simulink model "ISRTest2"  (Simulink 6.6)
settings: Solver=ode3  StartTime=0.0  StopTime=time(end)  FixedStep=0.01  RelTol=1e-3
values from neighbouring files (symbols this model uses):
  apSampleTime = 0.01    [Load_Replay.m]    (also in loadReplayMay2013.m; loadTuneRollReplay_May2013.m)
undefined symbols (not defined in the file or in its folder): bankCommandLimit, fOrderingInOut, ISA_g, maxAcc, maxEta
libraries: simulink x14, aerolibconvert2 x11, dsPICdrivers x7, SLUGS_Library x3, dspmtrx3 x2, aerolibutil x1
(part 2 of 2)

== system ISRTest2/Get 2D Groundspeed/Norm/Subsystem1 ==
  x : Inport
  C Function Call : S-Function  Tag=dsPIC_dsPIC_CFunctionCall  FunctionName=dsPIC_C_function_Call  Parameters=INPUT_SIZE,OUTPUT_SIZE,InputType,OutputType,SampleTime,fOrderingInOut  mask(C Function Call){fctName='mySqrt', INPUT_SIZE=1, INPUT1=real32, INPUT2=--, INPUT3=--, OUTPUT_SIZE=1, OUTPUT1=real32, SampleTime=-1, InputType=[ 7 ], OutputType=[ 7 ], FctDeclaration=extern real32_T mySqrt(real32_T u1);, FctCall=%y1 = mySqrt(%u1);, OrderingInOutPopup=None}
      mask prompts: fctName "Function Name"; INPUT_SIZE "Global Input Size"; INPUT1 "Input 1"; INPUT2 "Input 2"; INPUT3 "Input 3"; OUTPUT_SIZE "Output size"; OUTPUT1 "Output type"; InputType "NbrInput"; OutputType "NbrOutput"; FctDeclaration "Function Declaration :"; FctCall "Function Call :"; OrderingInOutPopup "Block Ordering Input / Output"
      mask help: call user defined C function
      mask init:
      | dsPIC_C_function_Call_callback();
      mask Help: http://www.kerhuel.eu/wiki/index.php5?title=Block/C_Function_Call#1
      mask StyleString: edit,edit,popup(--|int8|uint8|int16|uint16|int32|uint32|real32|real64),popup(--|int8|uint8|int16|uint16|int32|uint32|real32|real64),popup(--|int8|uint8|int16|uint16|int32|uint32|real32|real64),edit,popup(--|int8|uint8|int16|uint16|int32|uint32|real32|real64),edit,edit,edit,edit,edit,popup(None|Input|Output|Input & Output)
      mask CallbackString:
      | dsPIC_C_function_Call_callback();|dsPIC_C_function_Call_callback();|dsPIC_C_function_Call_callback();|dsPIC_C_function_Call_callback();
      | |dsPIC_C_function_Call_callback();|dsPIC_C_function_Call_callback();|dsPIC_C_function_Call_callback();|dsPIC_C_function_Call_callback();|||% for information only|% for information only|
      mask Display:
      | fprintf('C function call\nmySqrt');
      | port_label('input',1,' u1');
      | port_label('output',1,'y');
  Environment Controller : Subsystem  mask(Environment Controller){}
      mask help: Output the simulation (Sim) or Real-Time Workshop (RTW) port depending on the current environment. With optimizations enabled, unnecessary blocks leading to the unused port are not executed. Both input signals must be the same width.
      mask init:
      | switch_mode = rtwenvironmentmode(bdroot(gcbh));
  Math Function1 : Math  Operator=sqrt  SaturateOnIntegerOverflow=on
  negprotect : Stateflow chart
  sqrt(x) : Outport
  wires:
  C Function Call/1 -> Environment Controller/2(RTW)
  Math Function1/1 -> Environment Controller/1(Sim)
  Environment Controller/1(Out) -> sqrt(x)/1
  negprotect/1(zpVal) -> C Function Call/1, Math Function1/1
  x/1 -> negprotect/1(val)

== system ISRTest2/L2+/Get Sin, Cos eta/2D Dot Product  ==
  Vxyz : Inport
  L2_vec : Inport  Port=2
  Demux : Demux  Outputs=3
  Demux1 : Demux  Outputs=3
  Product : Product  RndMeth=Zero
  Product1 : Product  RndMeth=Zero
  Subtract : Sum  Inputs=2  OutScaling=2^-10
  Terminator : Terminator
  Terminator1 : Terminator
  2D _dot : Outport
  wires:
  Vxyz/1 -> Demux/1
  Subtract/1 -> 2D _dot/1
  L2_vec/1 -> Demux1/1
  Product1/1 -> Subtract/2
  Product/1 -> Subtract/1
  Demux1/3 -> Terminator1/1
  Demux/3 -> Terminator/1
  Demux1/1 -> Product/1
  Demux/1 -> Product/2
  Demux1/2 -> Product1/1
  Demux/2 -> Product1/2

== system ISRTest2/L2+/Get Sin, Cos eta/Get  Groundspeed ==
  L2_vec : Inport  SampleTime=apSampleTime
  Norm : Subsystem
  Zero out Z1 : Stateflow chart
  |L2| : Outport
  wires:
  L2_vec/1 -> Zero out Z1/1(Pin)
  Zero out Z1/1(P) -> Norm/1(Vector)
  Norm/1(Norm) -> |L2|/1

== system ISRTest2/L2+/Get Sin, Cos eta/Get ZProd ==
  L2_vec : Inport
  Vxyz : Inport  Port=2
  Demux : Demux  Outputs=3
  Demux1 : Demux  Outputs=3
  Product : Product  RndMeth=Zero
  Product1 : Product  RndMeth=Zero
  Subtract : Sum  Inputs=+-  OutScaling=2^-10
  Terminator : Terminator
  Terminator1 : Terminator
  Z_prod : Outport
  wires:
  Demux/3 -> Terminator/1
  Demux1/3 -> Terminator1/1
  Demux/1 -> Product/2
  Demux1/2 -> Product/1
  Demux/2 -> Product1/2
  Demux1/1 -> Product1/1
  Product/1 -> Subtract/1
  Product1/1 -> Subtract/2
  L2_vec/1 -> Demux1/1
  Subtract/1 -> Z_prod/1
  Vxyz/1 -> Demux/1

== system ISRTest2/L2+/Subsystem/Subsystem2 ==
  x : Inport
  C Function Call : S-Function  Tag=dsPIC_dsPIC_CFunctionCall  AncestorBlock=dsPICdrivers/OTHERS/C Function Call  FunctionName=dsPIC_C_function_Call  Parameters=INPUT_SIZE,OUTPUT_SIZE,InputType,OutputType,SampleTime,fOrderingInOut  mask(C Function Call){fctName='myAtan', INPUT_SIZE=1, INPUT1=real32, INPUT2=--, INPUT3=--, OUTPUT_SIZE=1, OUTPUT1=real32, SampleTime=-1, InputType=[ 7 ], OutputType=[ 7 ], FctDeclaration=extern real32_T myAtan(real32_T u1);, FctCall=%y1 = myAtan(%u1);, OrderingInOutPopup=None}
      mask prompts: fctName "Function Name"; INPUT_SIZE "Global Input Size"; INPUT1 "Input 1"; INPUT2 "Input 2"; INPUT3 "Input 3"; OUTPUT_SIZE "Output size"; OUTPUT1 "Output type"; InputType "NbrInput"; OutputType "NbrOutput"; FctDeclaration "Function Declaration :"; FctCall "Function Call :"; OrderingInOutPopup "Block Ordering Input / Output"
      mask help: call user defined C function
      mask init:
      | dsPIC_C_function_Call_callback();
      mask Help: http://www.kerhuel.eu/wiki/index.php5?title=Block/C_Function_Call#1
      mask StyleString: edit,edit,popup(--|int8|uint8|int16|uint16|int32|uint32|real32|real64),popup(--|int8|uint8|int16|uint16|int32|uint32|real32|real64),popup(--|int8|uint8|int16|uint16|int32|uint32|real32|real64),edit,popup(--|int8|uint8|int16|uint16|int32|uint32|real32|real64),edit,edit,edit,edit,edit,popup(None|Input|Output|Input & Output)
      mask CallbackString:
      | dsPIC_C_function_Call_callback();|dsPIC_C_function_Call_callback();|dsPIC_C_function_Call_callback();|dsPIC_C_function_Call_callback();
      | |dsPIC_C_function_Call_callback();|dsPIC_C_function_Call_callback();|dsPIC_C_function_Call_callback();|dsPIC_C_function_Call_callback();|||% for information only|% for information only|
      mask Display:
      | fprintf('C function call\nmyAtan');
      | port_label('input',1,' u1');
      | port_label('output',1,'y');
  Environment Controller : Subsystem  AncestorBlock=|  mask(Environment Controller){}
      | simulink/Signal
      | Routing/Environment
      | Controller
      mask help: Output the simulation (Sim) or Real-Time Workshop (RTW) port depending on the current environment. With optimizations enabled, unnecessary blocks leading to the unused port are not executed. Both input signals must be the same width.
      mask init:
      | switch_mode = rtwenvironmentmode(bdroot(gcbh));
  Trigonometric Function : Trigonometry  Operator=atan
  atan(x) : Outport
  wires:
  x/1 -> C Function Call/1, Trigonometric Function/1
  Trigonometric Function/1 -> Environment Controller/1(Sim)
  C Function Call/1 -> Environment Controller/2(RTW)
  Environment Controller/1(Out) -> atan(x)/1

== system ISRTest2/L2+/Subsystem4/Environment Controller ==
  Sim : Inport
  RTW : Inport  Port=2
  Environment Switch : Switch  Criteria=u2 ~= 0  ZeroCross=off  InputSameDT=on
  Numerical Unity : SignalConversion  ConversionOutput=Bus copy
  Switch Control : Constant  Value=switch_mode  OutDataTypeMode=boolean
  Out : Outport
  wires:
  Numerical Unity/1 -> Out/1
  RTW/1 -> Environment Switch/3
  Environment Switch/1 -> Numerical Unity/1
  Switch Control/1 -> Environment Switch/2
  Sim/1 -> Environment Switch/1

== system ISRTest2/Point  Surveillance/P2CC Data/Norm1 ==
  Vector : Inport
  Subsystem1 : Subsystem  AncestorBlock=SLUGS_Library/Subsystem1
  Subsystem3 : Subsystem  AncestorBlock=SLUGS_Library/Subsystem3
  Norm : Outport
  wires:
  Subsystem3/1(x dot y) -> Subsystem1/1(x)
  Vector/1 -> Subsystem3/2(y), Subsystem3/1(x)
  Subsystem1/1(sqrt(x)) -> Norm/1

== system ISRTest2/Point  Surveillance/P2CC Data/Subsystem10 ==
  x : Inport
  Trigonometric Function : Trigonometry  Operator=acos
  acos(x) : Outport
  wires:
  x/1 -> Trigonometric Function/1
  Trigonometric Function/1 -> acos(x)/1

== system ISRTest2/Point  Surveillance/P2CC Data/Subsystem4 ==
  x : Inport
  y : Inport  Port=2
  Trigonometric Function : Trigonometry  Operator=atan2
  atan2(x,y) : Outport
  wires:
  Trigonometric Function/1 -> atan2(x,y)/1
  y/1 -> Trigonometric Function/2
  x/1 -> Trigonometric Function/1

== system ISRTest2/Camera Track/Norm/Subsystem1/Environment Controller ==
  Sim : Inport
  RTW : Inport  Port=2
  Environment Switch : Switch  Criteria=u2 ~= 0  ZeroCross=off  InputSameDT=on
  Numerical Unity : SignalConversion  ConversionOutput=Bus copy
  Switch Control : Constant  Value=switch_mode  OutDataTypeMode=boolean
  Out : Outport
  wires:
  Numerical Unity/1 -> Out/1
  RTW/1 -> Environment Switch/3
  Environment Switch/1 -> Numerical Unity/1
  Switch Control/1 -> Environment Switch/2
  Sim/1 -> Environment Switch/1

== system ISRTest2/Camera Track/Norm1/Subsystem1/Environment Controller ==
  Sim : Inport
  RTW : Inport  Port=2
  Environment Switch : Switch  Criteria=u2 ~= 0  ZeroCross=off  InputSameDT=on
  Numerical Unity : SignalConversion  ConversionOutput=Bus copy
  Switch Control : Constant  Value=switch_mode  OutDataTypeMode=boolean
  Out : Outport
  wires:
  Sim/1 -> Environment Switch/1
  Switch Control/1 -> Environment Switch/2
  Environment Switch/1 -> Numerical Unity/1
  RTW/1 -> Environment Switch/3
  Numerical Unity/1 -> Out/1

== system ISRTest2/Get 2D Groundspeed/Norm/Subsystem1/Environment Controller ==
  Sim : Inport
  RTW : Inport  Port=2
  Environment Switch : Switch  Criteria=u2 ~= 0  ZeroCross=off  InputSameDT=on
  Numerical Unity : SignalConversion  ConversionOutput=Bus copy
  Switch Control : Constant  Value=switch_mode  OutDataTypeMode=boolean
  Out : Outport
  wires:
  Sim/1 -> Environment Switch/1
  Switch Control/1 -> Environment Switch/2
  Environment Switch/1 -> Numerical Unity/1
  RTW/1 -> Environment Switch/3
  Numerical Unity/1 -> Out/1

== system ISRTest2/L2+/Get Sin, Cos eta/Get  Groundspeed/Norm ==
  Vector : Inport
  Subsystem1 : Subsystem  AncestorBlock=SLUGS_Library/Subsystem1
  Subsystem3 : SLUGS_Library/Subsystem3  SystemSampleTime=-1
  Norm : Outport
  wires:
  Subsystem1/1(sqrt(x)) -> Norm/1
  Vector/1 -> Subsystem3/1, Subsystem3/2
  Subsystem3/1 -> Subsystem1/1(x)

== system ISRTest2/L2+/Subsystem/Subsystem2/Environment Controller ==
  Sim : Inport
  RTW : Inport  Port=2
  Environment Switch : Switch  Criteria=u2 ~= 0  ZeroCross=off  InputSameDT=on
  Numerical Unity : SignalConversion  ConversionOutput=Bus copy
  Switch Control : Constant  Value=switch_mode  OutDataTypeMode=boolean
  Out : Outport
  wires:
  Numerical Unity/1 -> Out/1
  RTW/1 -> Environment Switch/3
  Environment Switch/1 -> Numerical Unity/1
  Switch Control/1 -> Environment Switch/2
  Sim/1 -> Environment Switch/1

== system ISRTest2/Point  Surveillance/P2CC Data/Norm1/Subsystem1 ==
  x : Inport
  Math Function : Math  Operator=sqrt  SaturateOnIntegerOverflow=on
  negprotect : Stateflow chart
  sqrt(x) : Outport
  wires:
  Math Function/1 -> sqrt(x)/1
  negprotect/1(zpVal) -> Math Function/1
  x/1 -> negprotect/1(val)

== system ISRTest2/Point  Surveillance/P2CC Data/Norm1/Subsystem3 ==
  x : Inport
  y : Inport  Port=2
  Embedded MATLAB Function : Stateflow chart
  x dot y : Outport
  wires:
  y/1 -> Embedded MATLAB Function/2(y)
  x/1 -> Embedded MATLAB Function/1(x)
  Embedded MATLAB Function/1(xDoty) -> x dot y/1

== system ISRTest2/L2+/Get Sin, Cos eta/Get  Groundspeed/Norm/Subsystem1 ==
  x : Inport
  C Function Call : S-Function  Tag=dsPIC_dsPIC_CFunctionCall  FunctionName=dsPIC_C_function_Call  Parameters=INPUT_SIZE,OUTPUT_SIZE,InputType,OutputType,SampleTime,fOrderingInOut  mask(C Function Call){fctName='mySqrt', INPUT_SIZE=1, INPUT1=real32, INPUT2=--, INPUT3=--, OUTPUT_SIZE=1, OUTPUT1=real32, SampleTime=-1, InputType=[ 7 ], OutputType=[ 7 ], FctDeclaration=extern real32_T mySqrt(real32_T u1);, FctCall=%y1 = mySqrt(%u1);, OrderingInOutPopup=None}
      mask prompts: fctName "Function Name"; INPUT_SIZE "Global Input Size"; INPUT1 "Input 1"; INPUT2 "Input 2"; INPUT3 "Input 3"; OUTPUT_SIZE "Output size"; OUTPUT1 "Output type"; InputType "NbrInput"; OutputType "NbrOutput"; FctDeclaration "Function Declaration :"; FctCall "Function Call :"; OrderingInOutPopup "Block Ordering Input / Output"
      mask help: call user defined C function
      mask init:
      | dsPIC_C_function_Call_callback();
      mask Help: http://www.kerhuel.eu/wiki/index.php5?title=Block/C_Function_Call#1
      mask StyleString: edit,edit,popup(--|int8|uint8|int16|uint16|int32|uint32|real32|real64),popup(--|int8|uint8|int16|uint16|int32|uint32|real32|real64),popup(--|int8|uint8|int16|uint16|int32|uint32|real32|real64),edit,popup(--|int8|uint8|int16|uint16|int32|uint32|real32|real64),edit,edit,edit,edit,edit,popup(None|Input|Output|Input & Output)
      mask CallbackString:
      | dsPIC_C_function_Call_callback();|dsPIC_C_function_Call_callback();|dsPIC_C_function_Call_callback();|dsPIC_C_function_Call_callback();
      | |dsPIC_C_function_Call_callback();|dsPIC_C_function_Call_callback();|dsPIC_C_function_Call_callback();|dsPIC_C_function_Call_callback();|||% for information only|% for information only|
      mask Display:
      | fprintf('C function call\nmySqrt');
      | port_label('input',1,' u1');
      | port_label('output',1,'y');
  Environment Controller : Subsystem  mask(Environment Controller){}
      mask help: Output the simulation (Sim) or Real-Time Workshop (RTW) port depending on the current environment. With optimizations enabled, unnecessary blocks leading to the unused port are not executed. Both input signals must be the same width.
      mask init:
      | switch_mode = rtwenvironmentmode(bdroot(gcbh));
  Math Function1 : Math  Operator=sqrt  SaturateOnIntegerOverflow=on
  negprotect : Stateflow chart
  sqrt(x) : Outport
  wires:
  x/1 -> negprotect/1(val)
  negprotect/1(zpVal) -> Math Function1/1, C Function Call/1
  Environment Controller/1(Out) -> sqrt(x)/1
  Math Function1/1 -> Environment Controller/1(Sim)
  C Function Call/1 -> Environment Controller/2(RTW)

== system ISRTest2/L2+/Get Sin, Cos eta/Get  Groundspeed/Norm/Subsystem1/Environment Controller ==
  Sim : Inport
  RTW : Inport  Port=2
  Environment Switch : Switch  Criteria=u2 ~= 0  ZeroCross=off  InputSameDT=on
  Numerical Unity : SignalConversion  ConversionOutput=Bus copy
  Switch Control : Constant  Value=switch_mode  OutDataTypeMode=boolean
  Out : Outport
  wires:
  Numerical Unity/1 -> Out/1
  RTW/1 -> Environment Switch/3
  Environment Switch/1 -> Numerical Unity/1
  Switch Control/1 -> Environment Switch/2
  Sim/1 -> Environment Switch/1

== matlab function Zero out Z1 ==
  data: P output inherited; Pin input inherited
function P = P2D(Pin)
% This block supports an embeddable subset of the MATLAB language.
% See the help menu for details. 

P = [Pin(1); Pin(2); 0];

== matlab function L2+/Get Sin, Cos eta/Get Groundspeed/Norm/Subsystem1/negprotect ==
  data: val input inherited; zpVal output inherited
function zpVal = negProt(val)
% This block supports an embeddable subset of the MATLAB language.
% See the help menu for details. 

if val >= single(0.0001)
    zpVal = val;
else
    zpVal = single(0.0001);
end

== matlab function Camera Track/Euler Angles to Direction Cosine Matrix/Subsystem5/myMux Fun2 ==
  data: u1 input inherited; y output inherited; u2 input inherited; u3 input inherited
function y = myMux3(u1, u2, u3)
% This block supports an embeddable subset of the MATLAB language.
% See the help menu for details. 

y = [u1(1); u2(1); u3(1)];

== matlab function L2+/Get Sin, Cos eta/Get Groundspeed/Zero out Z1 ==
  data: P output inherited; Pin input inherited
function P = P2D(Pin)
% This block supports an embeddable subset of the MATLAB language.
% See the help menu for details. 

P = [Pin(1); Pin(2); 0];

== matlab function Camera Track/Norm1/Subsystem1/negprotect ==
  data: val input inherited; zpVal output inherited
function zpVal = negProt(val)
% This block supports an embeddable subset of the MATLAB language.
% See the help menu for details. 

if val >= single(0.0001)
    zpVal = val;
else
    zpVal = single(0.0001);
end

== matlab function Camera Track/Norm1/Subsystem3/Embedded MATLAB Function ==
  data: x input inherited; y input inherited; xDoty output inherited
function xDoty = myDot(x,y)
% This block supports an embeddable subset of the MATLAB language.
% See the help menu for details. 

xDoty = x(1)*y(1) + x(2)*y(2) + x(3)*y(3);

== matlab function Get 2D Groundspeed/Norm/Subsystem1/negprotect ==
  data: val input inherited; zpVal output inherited
function zpVal = negProt(val)
% This block supports an embeddable subset of the MATLAB language.
% See the help menu for details. 

if val >= single(0.0001)
    zpVal = val;
else
    zpVal = single(0.0001);
end

== matlab function Camera Track/Euler Angles to Direction Cosine Matrix/Create Transformation Matrix/myMux Fun1 ==
  data: u1 input inherited; y output inherited; u2 input inherited; u3 input inherited; u4 input inherited; u5 input inherited; u6 input inherited; u7 input inherited; u8 input inherited; u9 input inherited
function y = myMux3(u1, u2, u3, u4, u5, u6, u7, u8, u9)
% This block supports an embeddable subset of the MATLAB language.
% See the help menu for details. 

y = [u1(1); u2(1); u3(1);u4(1); u5(1); u6(1); u7(1); u8(1); u9(1)];

== matlab function Camera Track/Euler Angles to Direction Cosine Matrix/Subsystem5/myMux Fun1 ==
  data: u1 input inherited; y output inherited; u2 input inherited; u3 input inherited
function y = myMux3(u1, u2, u3)
% This block supports an embeddable subset of the MATLAB language.
% See the help menu for details. 

y = [u1(1); u2(1); u3(1)];

== matlab function Point Surveillance/P2CC Data/Norm1/Subsystem1/negprotect ==
  data: val input inherited; zpVal output inherited
function zpVal = negProt(val)
% This block supports an embeddable subset of the MATLAB language.
% See the help menu for details. 

if val >= single(0.0001)
    zpVal = val;
else
    zpVal = single(0.0001);
end

== matlab function Point Surveillance/P2CC Data/Norm1/Subsystem3/Embedded MATLAB Function ==
  data: x input inherited; y input inherited; xDoty output inherited
function xDoty = myDot(x,y)
% This block supports an embeddable subset of the MATLAB language.
% See the help menu for details. 

xDoty = x(1)*y(1) + x(2)*y(2) + x(3)*y(3);

== matlab function Point Surveillance/P2CC Data/negprotect1 ==
  data: val input inherited; zpVal output inherited
function zpVal = negProt(val)
% This block supports an embeddable subset of the MATLAB language.
% See the help menu for details. 

if val >= single(0.0001)
    zpVal = val;
else
    zpVal = single(0.0001);
end

== matlab function Point Surveillance/P2CC Data/negprotect2 ==
  data: val input inherited; zpVal output inherited
function zpVal = negProt(val)
% This block supports an embeddable subset of the MATLAB language.
% See the help menu for details. 

if val >= single(0.0001)
    zpVal = val;
else
    zpVal = single(0.0001);
end

== matlab function L2+/Get Sin, Cos eta/negprotect ==
  data: val input inherited; zpVal output inherited
function zpVal = negProt(val)
% This block supports an embeddable subset of the MATLAB language.
% See the help menu for details. 

if val >= single(0.0001)
    zpVal = val;
else
    zpVal = single(0.0001);
end

== matlab function L2+/L2+/negprotect ==
  data: val input inherited; zpVal output inherited
function zpVal = negProt(val)
% This block supports an embeddable subset of the MATLAB language.
% See the help menu for details. 

if val >= single(0.0001)
    zpVal = val;
else
    zpVal = single(0.0001);
end

== matlab function Point Surveillance/myMux Fun2 ==
  data: u1 input inherited; y output inherited; u2 input inherited; u3 input inherited
function y = myMux(u1, u2, u3)
% This block supports an embeddable subset of the MATLAB language.
% See the help menu for details. 

y = [u1(1); u2(1); u3(1)];

== matlab function Camera Track/Norm/Subsystem1/negprotect ==
  data: val input inherited; zpVal output inherited
function zpVal = negProt(val)
% This block supports an embeddable subset of the MATLAB language.
% See the help menu for details. 

if val >= single(0.0001)
    zpVal = val;
else
    zpVal = single(0.0001);
end

== matlab function Zero out Z3 ==
  data: P output inherited; Pin input inherited
function P = P2D(Pin)
% This block supports an embeddable subset of the MATLAB language.
% See the help menu for details. 

P = [Pin(1); Pin(2); 0];

== matlab function Zero out Z2 ==
  data: P output inherited; Pin input inherited
function P = P2D(Pin)
% This block supports an embeddable subset of the MATLAB language.
% See the help menu for details. 

P = [Pin(1); Pin(2); 0];

== matlab function Camera Track/Norm/Subsystem3/Embedded MATLAB Function ==
  data: x input inherited; y input inherited; xDoty output inherited
function xDoty = myDot(x,y)
% This block supports an embeddable subset of the MATLAB language.
% See the help menu for details. 

xDoty = x(1)*y(1) + x(2)*y(2) + x(3)*y(3);
